simulink model "sampleModel1986"  (R2023a)
settings: Solver=VariableStepAuto  StartTime=0.0  StopTime=10.0  RelTol=1e-3
libraries: hdlsllib x5, simulink x1
settings Model: Creator=user1  LastModifiedBy=user1

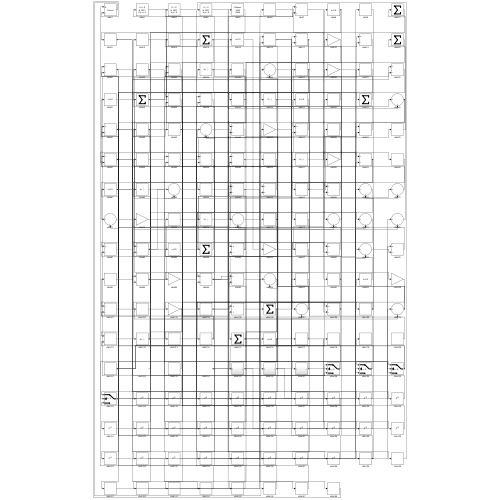
[thumbnail: Simulink's stored preview of the top-level diagram]
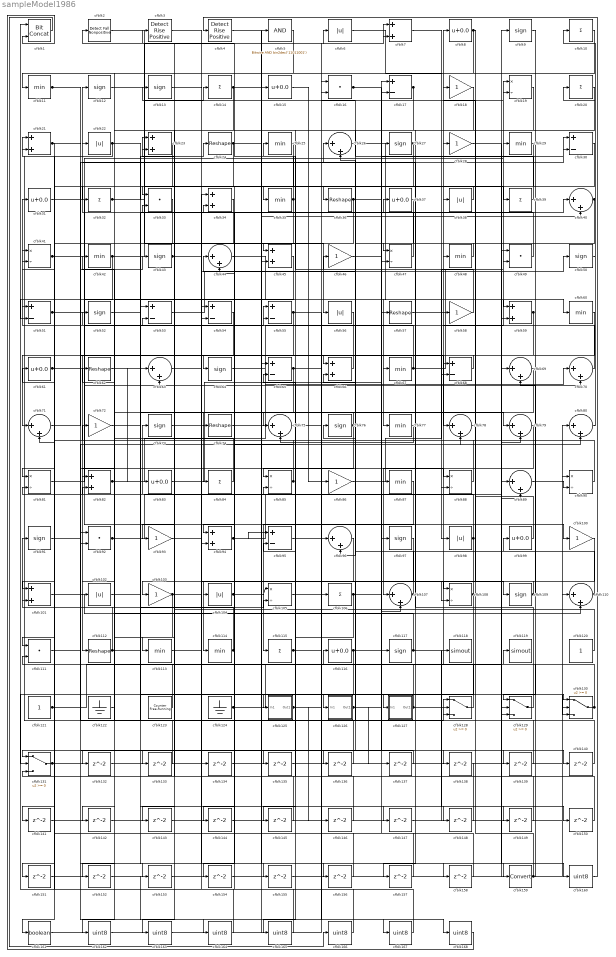
== system sampleModel1986 ==
  cfblk1 : hdlsllib/Logic and Bit Operations/Bit Concat  numInputs=2
  cfblk{10,14,20,32,39,84,106,115} (8 alike) : Sum  Inputs=+
  cfblk{18,28,46,58,72,86,93,100,103} (9 alike) : Gain
  cfblk{7,21,23,34,45,59,66,82,94,101} (10 alike) : Sum
  cfblk{6,22,38,56,98,102,104} (7 alike) : Abs  SaturateOnIntegerOverflow=off
  cfblk{19,41,47,81,85,88,90,105,108} (9 alike) : Product  Inputs=*/  RndMeth=Zero  SaturateOnIntegerOverflow=on
  cfblk{26,40,44,63,69..71,75,78..80,89,96,107,110} (15 alike) : Sum  Inputs=|++
  cfblk{9,12..13,27,43,50,52,64,73,76,91,97,109,117} (14 alike) : Signum
  cfblk{11,25,29,35,42,48,60,67,77,87,113..114} (12 alike) : MinMax
  cfblk{16,33,49,92,111} (5 alike) : DotProduct  OutDataTypeStr=Inherit: Inherit via internal rule
  cfblk{24,36,57,62,74,112} (6 alike) : Reshape
  cfblk{8,15,31,37,61,83,99,116} (8 alike) : Bias  Bias=0.0  SaturateOnIntegerOverflow=off
  cfblk118 : ToWorkspace  VariableName=simout  SaveFormat=Timeseries  SampleTime=-1
  cfblk119 : ToWorkspace  VariableName=simout  SaveFormat=Timeseries  SampleTime=-1
  cfblk120 : Constant  SampleTime=-1
  cfblk121 : Constant  SampleTime=-1
  cfblk122 : Ground
  cfblk123 : hdlsllib/Sources/Counter Free-Running  NumBits=16  tsamp=-1
  cfblk124 : Ground
  cfblk125 : Subsystem
      settings: LibrarySourceBlock=|
      | hdlsllib/Ports &
      | Subsystems/Subsystem
  cfblk126 : Subsystem
      settings: LibrarySourceBlock=|
      | hdlsllib/Ports &
      | Subsystems/Subsystem
  cfblk127 : Subsystem
      settings: LibrarySourceBlock=|
      | hdlsllib/Ports &
      | Subsystems/Subsystem
  cfblk{128..131} (4 alike) : Switch  SaturateOnIntegerOverflow=off  InputSameDT=off
  cfblk{132..158} (27 alike) : Delay  SampleTime=1
  cfblk159 : DataTypeConversion  SaturateOnIntegerOverflow=off  RndMeth=Floor
  cfblk{160,162..168} (8 alike) : DataTypeConversion  OutDataTypeStr=uint8  SaturateOnIntegerOverflow=off  RndMeth=Floor
  cfblk161 : DataTypeConversion  OutDataTypeStr=boolean  SaturateOnIntegerOverflow=off  RndMeth=Floor
  cfblk{17,30,51,53..55,65,68,95} (9 alike) : Sum  Inputs=+-
  cfblk2 : hdlsllib/Logic and Bit Operations/Detect Fall Nonpositive  vinit=0  OutDataTypeStr=boolean
  cfblk3 : hdlsllib/Logic and Bit Operations/Detect Rise Positive  vinit=0  OutDataTypeStr=boolean
  cfblk4 : hdlsllib/Logic and Bit Operations/Detect Rise Positive  vinit=0  OutDataTypeStr=boolean
  cfblk5 : simulink/Logic and Bit Operations/Bitwise Operator  logicop=AND  UseBitMask=on  BitMask=bin2dec('11011001')  BitMaskRealWorld=Stored Integer
      settings: LibrarySourceBlock=|
      | hdlsllib/Logic and Bit
      | Operations/Bitwise
      | Operator
  wires:
  cfblk15/1 -> cfblk86/1
  cfblk37/1 -> cfblk73/1
  cfblk70/1 -> cfblk8/1
  cfblk108/1 -> cfblk103/1, cfblk161/1
  cfblk68/1 -> cfblk64/1
  cfblk81/1 -> cfblk55/1
  cfblk130/1 -> cfblk76/1, cfblk95/2
  cfblk32/1 -> cfblk14/1, cfblk24/1
  cfblk105/1 -> cfblk106/1
  cfblk121/1 -> cfblk48/1, cfblk69/1, cfblk45/2
  cfblk128/1 -> cfblk116/1
  cfblk74/1 -> cfblk70/1
  cfblk79/1 -> cfblk107/1
  cfblk59/1 -> cfblk112/1, cfblk87/1
  cfblk63/1 -> cfblk50/1
  cfblk31/1 -> cfblk100/1
  cfblk95/1 -> cfblk127/1(In1)
  cfblk51/1 -> cfblk70/2, cfblk153/1
  cfblk55/1 -> cfblk94/1, cfblk149/1
  cfblk7/1 -> cfblk98/1
  cfblk80/1 -> cfblk20/1
  cfblk35/1 -> cfblk2/1, cfblk111/1
  cfblk82/1 -> cfblk19/1, cfblk63/1
  cfblk4/1 -> cfblk159/1
  cfblk90/1 -> cfblk72/1
  cfblk107/1 -> cfblk53/2, cfblk81/2
  cfblk10/1 -> cfblk11/1
  cfblk75/1 -> cfblk19/2
  cfblk61/1 -> cfblk29/1, cfblk30/2
  cfblk8/1 -> cfblk108/1, cfblk152/1
  cfblk22/1 -> cfblk128/1, cfblk63/2
  cfblk120/1 -> cfblk83/1
  cfblk67/1 -> cfblk9/1, cfblk3/1
  cfblk112/1 -> cfblk91/1, cfblk105/2
  cfblk52/1 -> cfblk40/1
  cfblk47/1 -> cfblk12/1
  cfblk99/1 -> cfblk18/1
  cfblk66/1 -> cfblk31/1
  cfblk56/1 -> cfblk55/2
  cfblk83/1 -> cfblk15/1
  cfblk42/1 -> cfblk6/1, cfblk51/2
  cfblk71/1 -> cfblk43/1
  cfblk21/1 -> cfblk141/1, cfblk164/1
  cfblk46/1 -> cfblk117/1
  cfblk54/1 -> cfblk71/1
  cfblk26/1 -> cfblk59/1
  cfblk44/1 -> cfblk77/1
  cfblk2/1 -> cfblk39/1
  cfblk87/1 -> cfblk115/1
  cfblk17/1 -> cfblk96/2, cfblk45/1
  cfblk84/1 -> cfblk62/1
  cfblk60/1 -> cfblk78/1
  cfblk89/1 -> cfblk90/2
  cfblk18/1 -> cfblk85/1
  cfblk124/1 -> cfblk107/2, cfblk128/3
  cfblk38/1 -> cfblk35/1
  cfblk110/1 -> cfblk44/1, cfblk99/1
  cfblk65/1 -> cfblk82/1, cfblk108/2
  cfblk12/1 -> cfblk56/1
  cfblk103/1 -> cfblk109/1, cfblk142/1
  cfblk101/1 -> cfblk110/2
  cfblk48/1 -> cfblk47/1
  cfblk122/1 -> cfblk52/1
  cfblk29/1 -> cfblk101/1
  cfblk40/1 -> cfblk129/3, cfblk157/1
  cfblk6/1 -> cfblk58/1
  cfblk58/1 -> cfblk25/1
  cfblk45/1 -> cfblk102/1
  cfblk33/1 -> cfblk92/2
  cfblk30/1 -> cfblk113/1
  cfblk98/1 -> cfblk126/1(In1), cfblk65/2
  cfblk88/1 -> cfblk21/1
  cfblk93/1 -> cfblk37/1
  cfblk23/1 -> cfblk32/1
  cfblk3/1 -> cfblk36/1
  cfblk53/1 -> cfblk17/2
  cfblk50/1 -> cfblk10/1
  cfblk106/1 -> cfblk27/1, cfblk125/1(In1), cfblk145/1
  cfblk92/1 -> cfblk49/1, cfblk130/3
  cfblk36/1 -> cfblk30/1, cfblk74/1
  cfblk20/1 -> cfblk67/1
  cfblk85/1 -> cfblk41/1, cfblk44/2
  cfblk64/1 -> cfblk66/1
  cfblk123/1 -> cfblk21/2
  cfblk27/1 -> cfblk143/1, cfblk144/1
  cfblk104/1 -> cfblk105/1, cfblk78/2
  cfblk43/1 -> cfblk93/1, cfblk88/2
  cfblk96/1 -> cfblk114/1
  cfblk115/1 -> cfblk130/1, cfblk7/1
  cfblk127/1(Out1) -> cfblk118/1, cfblk66/2
  cfblk78/1 -> cfblk28/1
  cfblk114/1 -> cfblk23/1, cfblk51/1
  cfblk39/1 -> cfblk13/1
  cfblk16/1 -> cfblk68/1, cfblk140/1
  cfblk69/1 -> cfblk84/1
  cfblk11/1 -> cfblk88/1, cfblk139/1
  cfblk76/1 -> cfblk75/1, cfblk165/1
  cfblk9/1 -> cfblk129/1
  cfblk77/1 -> cfblk75/2
  cfblk126/1(Out1) -> cfblk137/1, cfblk138/1
  cfblk94/1 -> cfblk57/1, cfblk95/1, cfblk7/2
  cfblk57/1 -> cfblk60/1
  cfblk73/1 -> cfblk47/2
  cfblk116/1 -> cfblk131/2, cfblk111/2, cfblk130/2, cfblk46/1, cfblk154/1
  cfblk41/1 -> cfblk89/1, cfblk68/2
  cfblk91/1 -> cfblk80/2
  cfblk49/1 -> cfblk26/2
  cfblk131/1 -> cfblk97/1, cfblk54/2
  cfblk117/1 -> cfblk42/1, cfblk150/1
  cfblk109/1 -> cfblk104/1, cfblk69/2
  cfblk129/1 -> cfblk22/1
  cfblk72/1 -> cfblk79/1
  cfblk24/1 -> cfblk81/1, cfblk40/2
  cfblk86/1 -> cfblk49/2
  cfblk125/1(Out1) -> cfblk146/1, cfblk147/1
  cfblk14/1 -> cfblk33/1, cfblk156/1
  cfblk19/1 -> cfblk132/1
  cfblk132/1 -> cfblk110/1
  cfblk97/1 -> cfblk133/1
  cfblk133/1 -> cfblk92/1
  cfblk13/1 -> cfblk134/1
  cfblk134/1 -> cfblk59/2
  cfblk111/1 -> cfblk135/1
  cfblk100/1 -> cfblk136/1
  cfblk136/1 -> cfblk53/1
  cfblk137/1 -> cfblk131/1
  cfblk138/1 -> cfblk131/3
  cfblk139/1 -> cfblk26/1
  cfblk140/1 -> cfblk82/2
  cfblk141/1 -> cfblk65/1
  cfblk142/1 -> cfblk80/1
  cfblk143/1 -> cfblk94/2
  cfblk144/1 -> cfblk128/2
  cfblk145/1 -> cfblk33/2
  cfblk146/1 -> cfblk71/2
  cfblk147/1 -> cfblk89/2
  cfblk62/1 -> cfblk148/1
  cfblk148/1 -> cfblk54/1
  cfblk149/1 -> cfblk85/2
  cfblk150/1 -> cfblk23/2
  cfblk25/1 -> cfblk151/1
  cfblk151/1 -> cfblk96/1
  cfblk153/1 -> cfblk79/2
  cfblk154/1 -> cfblk129/2
  cfblk113/1 -> cfblk155/1
  cfblk155/1 -> cfblk90/1
  cfblk156/1 -> cfblk41/2
  cfblk157/1 -> cfblk101/2
  cfblk102/1 -> cfblk158/1
  cfblk158/1 -> cfblk17/1
  cfblk159/1 -> cfblk38/1, cfblk119/1
  cfblk28/1 -> cfblk160/1
  cfblk160/1 -> cfblk4/1
  cfblk161/1 -> cfblk5/1
  cfblk5/1 -> cfblk162/1
  cfblk162/1 -> cfblk16/1
  cfblk34/1 -> cfblk163/1
  cfblk163/1 -> cfblk16/2
  cfblk164/1 -> cfblk34/1
  cfblk165/1 -> cfblk34/2
  cfblk1/1 -> cfblk166/1
  cfblk166/1 -> cfblk61/1
  cfblk152/1 -> cfblk167/1
  cfblk167/1 -> cfblk1/1
  cfblk135/1 -> cfblk168/1
  cfblk168/1 -> cfblk1/2

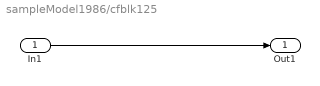
== system sampleModel1986/cfblk125 ==
  In1 : Inport
  Out1 : Outport
  wires:
  In1/1 -> Out1/1

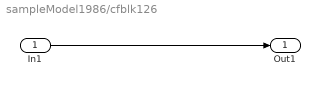
== system sampleModel1986/cfblk126 ==
  In1 : Inport
  Out1 : Outport
  wires:
  In1/1 -> Out1/1

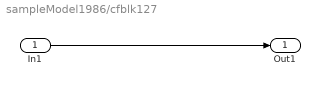
== system sampleModel1986/cfblk127 ==
  In1 : Inport
  Out1 : Outport
  wires:
  In1/1 -> Out1/1
